simulink model "Quadcopter_Dynamics_ver2"  (R2026a)
settings: Solver=VariableStepAuto  StopTime=20.0
libraries: slpidlib x1
settings Model: Creator=aarus  LastModifiedBy=Ashwini

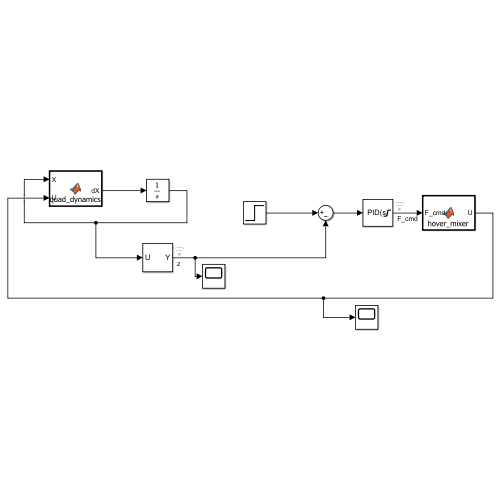
[thumbnail: Simulink's stored preview of the top-level diagram]
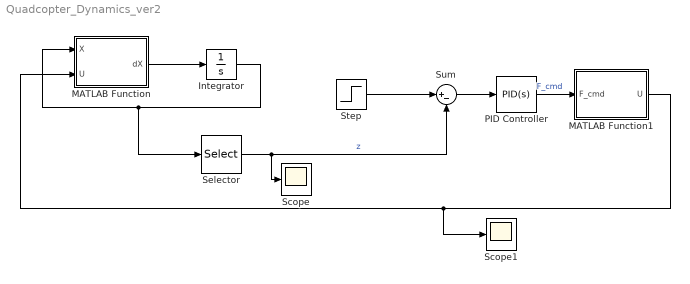
== system Quadcopter_Dynamics_ver2 ==
  Integrator : Integrator  InitialCondition=[0;0;0;0;0;0;0;0;0;0;0;0]
  MATLAB Function : MATLAB Function  TreatAsAtomicUnit=on
  MATLAB Function1 : MATLAB Function  TreatAsAtomicUnit=on
  PID Controller : slpidlib/PID Controller  Controller=PID  Form=Parallel  TimeDomain=Continuous-time  UseExternalTs=off  SampleTime=-1  IntegratorMethod=Forward Euler  FilterMethod=Forward Euler  ControllerParametersSource=internal  P=56.8136  I=7.3365  UseKiTs=off  D=31.7435  UseExternalDerivativeSource=off  N=100  UseFilter=on  TunerSelectOption=Transfer Function Based (PID Tuner App)  InitialConditionSource=internal  InitialConditionForIntegrator=0  InitialConditionForFilter=0  DifferentiatorICPrevScaledInput=0  ExternalReset=none  TrackingMode=off  Kt=1  LimitOutput=on  SatLimitsSource=internal  UpperSaturationLimit=20  LowerSaturationLimit=0  LinearizeAsGain=on  AntiWindupMode=none  Kb=1  LimitIntegrator=off  UpperIntegratorSaturationLimit=inf  LowerIntegratorSaturationLimit=-inf  POutMin=[]  POutMax=[]  IOutMin=[]  IOutMax=[]  DOutMin=[]  DOutMax=[]  NOutMin=[]  NOutMax=[]  SumOutMin=[]  SumOutMax=[]  SaturationOutMin=[]  SaturationOutMax=[]  PParamMin=[]  PParamMax=[]  IParamMin=[]  IParamMax=[]  DParamMin=[]  DParamMax=[]  NParamMin=[]  NParamMax=[]  KbParamMin=[]  KbParamMax=[]  KtParamMin=[]  KtParamMax=[]  KbOutMin=[]  KbOutMax=[]  KtOutMin=[]  KtOutMax=[]  IntegratorOutMin=[]  IntegratorOutMax=[]  FilterOutMin=[]  FilterOutMax=[]  SumI1OutMin=[]  SumI1OutMax=[]  SumI2OutMin=[]  SumI2OutMax=[]  SumI3OutMin=[]  SumI3OutMax=[]  SumI4OutMin=[]  SumI4OutMax=[]  SumDOutMin=[]  SumDOutMax=[]  DifferentiatorOutMin=[]  DifferentiatorOutMax=[]  FilterDiffOutCoefMin=[]  FilterDiffOutCoefMax=[]  ReciprocalOutMin=[]  ReciprocalOutMax=[]  SumDenOutMin=[]  SumDenOutMax=[]  SumNumOutMin=[]  SumNumOutMax=[]  DivideOutMin=[]  DivideOutMax=[]  UdiffTsProdOutMin=[]  UdiffTsProdOutMax=[]  NTsProdOutMin=[]  NTsProdOutMax=[]  UintegralTsProdOutMin=[]  UintegralTsProdOutMax=[]  UngainTsProdOutMin=[]  UngainTsProdOutMax=[]  ClampingZeroOutDataTypeStr=Inherit: Inherit via back propagation  ClampingZeroOutMin=[]  ClampingZeroOutMax=[]  FilterDenConstantOutDataTypeStr=Inherit: Inherit via back propagation  FilterDenConstantOutMin=[]  FilterDenConstantOutMax=[]  PCopyOutDataTypeStr=Inherit: Inherit via back propagation  PCopyOutMin=[]  PCopyOutMax=[]  NCopyOutDataTypeStr=Inherit: Inherit via back propagation  NCopyOutMin=[]  NCopyOutMax=[]  IntegratorContinuousStateAttributes=''  IntegratorStateMustResolveToSignalObject=off  IntegratorRTWStateStorageClass=Auto  FilterContinuousStateAttributes=''  FilterStateMustResolveToSignalObject=off  FilterRTWStateStorageClass=Auto  ParallelPVariant=InternalParameters  IdealPVariant=Disabled  IVariant=InternalParameters  DVariant=InternalParameters  IntegratorVariant=Continuous  SatVariant=Enabled  AWVariant=Passthrough  PCopyVariant=Disabled  TRVariant=Disabled  FdbkBlocksVariant=Forward  IdealPFdbkVariant=Disabled  SatFdbkVariant=Disabled  DerivativeFilterVariant=ContFilter  NVariant=InternalParameters  NCopyVariant=Disabled  FilterICVariant=InternalICsFilter  IntegratorICVariant=InternalICs  ExternalResetVariant=Disabled  TRSumVariant=Passthrough  SumFdbkVariant=Disabled  SumVariant=Sum_PID  TsampFilterVariant=InternalTs  TsampNgainVariant=Passthrough  TsampIntegralVariant=Disabled_SignalSpec  ExternalSaturationOutDataTypeStr=Inherit: Same as second input  DerivativeSourceVariant=ErrorSignal  PreIntVariant=InternalPreInt
  Scope : Scope
      settings: ActiveDisplayYMinimum=0  ActiveDisplayYMaximum=3
  Scope1 : Scope
      settings: ActiveDisplayYMinimum=-161.48199666525053  ActiveDisplayYMaximum=10000
  Selector : Selector  InputPortWidth=12  IndexOptions=Index vector (dialog)  Indices=5  OutputSizes=1
  Step : Step  Time=0  FinalValue=2  SampleTime=0
  Sum : Sum  Inputs=|+-
  wires:
  MATLAB Function/1(dX) -> Integrator/1
  Integrator/1 -> Selector/1, MATLAB Function/1(X)
  Selector/1 -> Scope/1, Sum/2  "z"
  Step/1 -> Sum/1
  Sum/1 -> PID Controller/1
  PID Controller/1 -> MATLAB Function1/1(F_cmd)  "F_cmd"
  MATLAB Function1/1(U) -> Scope1/1, MATLAB Function/2(U)

== matlab function Quadcopter_Dynamics_ver2/MATLAB Function ==
  data: X input; dX output; U input
function dX = quad_dynamics(X, U)
    % X: 12x1 state vector [x; x_dot; y; y_dot; z; z_dot; phi; phi_dot; theta; theta_dot; psi; psi_dot]
    % U: 4x1 control input vector [w1; w2; w3; w4] (rotor speeds in rad/s)
    
    % Table 1 Parameters
    m = 0.516; g = 9.81; l = 0.225; 
    Ixx = 4.984e-3; Iyy = 4.984e-3; Izz = 8.958e-3; 
    k = 2.996e-6; 
    b = 1.260e-7; 
    
    % Aerodynamic damping coefficients
    % Set to zero for ideal kinematics as numerical values are absent from Table 1
    Ax = 0; Ay = 0; Az = 0; 
    
    % Extract rotor speeds
    w1 = U(1); w2 = U(2); w3 = U(3); w4 = U(4);
    
    % Rotor-to-Force Mapping[cite: 2]
    F = k * (w1^2 + w2^2 + w3^2 + w4^2);
    tau_phi = l * k * (w4^2 - w2^2);
    tau_theta = l * k * (w3^2 - w1^2);
    tau_psi = b * (w1^2 - w2^2 + w3^2 - w4^2);
    
    tau_B = [tau_phi; tau_theta; tau_psi];

    % Extract states 
    x2 = X(2); x4 = X(4); x6 = X(6);
    phi = X(7); phi_dot = X(8); 
    theta = X(9); theta_dot = X(10); 
    psi = X(11); psi_dot = X(12);
    
    eta_dot = [phi_dot; theta_dot; psi_dot];
    
    % Trigonometric shorthands
    C_phi = cos(phi); S_phi = sin(phi);
    C_theta = cos(theta); S_theta = sin(theta);
    C_psi = cos(psi); S_psi = sin(psi);
    
    % Initialize output derivative vector
    dX = zeros(12,1);
    
    % Translational Equations
    dX(1) = x2;
    dX(2) = -(Ax/m)*x2 + (C_psi*S_theta*C_phi + S_psi*S_phi)*(F/m);
    dX(3) = x4;
    dX(4) = -(Ay/m)*x4 + (S_psi*S_theta*C_phi - C_psi*S_phi)*(F/m);
    
    % Z-axis with Ground Constraint
    z = X(5);
    z_ddot = -(Az/m)*x6 - g + (C_phi*C_theta)*(F/m);
    
    if z <= 0 && z_ddot < 0
        dX(5) = 0; % Hit the ground, velocity is 0
        dX(6) = 0; % Acceleration is 0
    else
        dX(5) = x6;
        dX(6) = z_ddot;
    end
    
    % Jacobian Matrix J(eta)[cite: 2]
    J11 = Ixx; J12 = 0; J13 = -Ixx*S_theta;
    J21 = 0; J22 = Iyy*C_phi^2 + Izz*S_phi^2; J23 = (Iyy - Izz)*C_phi*S_phi*C_theta;
    J31 = -Ixx*S_theta; J32 = (Iyy - Izz)*C_phi*S_phi*C_theta;
    J33 = Ixx*S_theta^2 + Iyy*S_phi^2*C_theta^2 + Izz*C_phi^2*C_theta^2;
    J = [J11 J12 J13; J21 J22 J23; J31 J32 J33];
    
    % Coriolis Matrix C(eta, eta_dot)
    C11 = 0;
    C12 = (Iyy - Izz)*(theta_dot*C_phi*S_phi + psi_dot*S_phi^2*C_theta) + (Izz - Iyy)*psi_dot*C_phi^2*C_theta - Ixx*psi_dot*C_theta;
    C13 = (Izz - Iyy)*psi_dot*C_phi*S_phi*C_theta^2;
    C21 = (Izz - Iyy)*(theta_dot*C_phi*S_phi + psi_dot*S_phi*C_theta) + (Iyy - Izz)*psi_dot*C_phi^2*C_theta + Ixx*psi_dot*C_theta;
    C22 = (Izz - Iyy)*phi_dot*C_phi*S_phi;
    C23 = -Ixx*psi_dot*S_theta*C_theta + Iyy*psi_dot*S_phi^2*S_theta*C_theta + Izz*psi_dot*C_phi^2*S_theta*C_theta;
    C31 = (Iyy - Izz)*psi_dot*C_theta^2*S_phi*C_phi - Ixx*theta_dot*C_theta;
    
    % Corrected C32 based on paper extraction
    C32 = (Izz - Iyy)*(theta_dot*C_phi*S_phi*S_theta + phi_dot*S_phi^2*C_theta) + (Iyy - Izz)*phi_dot*C_phi^2*C_theta + Ixx*psi_dot*S_theta*C_theta - Iyy*psi_dot*S_phi^2*S_theta*C_theta - Izz*psi_dot*C_phi^2*S_theta*C_theta;
    
    C33 = (Iyy - Izz)*phi_dot*C_phi*S_phi*C_theta^2 - Iyy*theta_dot*S_phi^2*C_theta*S_theta - Izz*theta_dot*C_phi^2*C_theta*S_theta + Ixx*theta_dot*C_theta*S_theta;
    C_mat = [C11 C12 C13; C21 C22 C23; C31 C32 C33];
    
    % Rotational Equations
    eta_ddot = J \ (tau_B - C_mat * eta_dot);
    
    dX(7) = phi_dot;
    dX(8) = eta_ddot(1);
    dX(9) = theta_dot;
    dX(10) = eta_ddot(2);
    dX(11) = psi_dot;
    dX(12) = eta_ddot(3);
end

== matlab function Quadcopter_Dynamics_ver2/MATLAB Function1 ==
  data: F_cmd input; U output
function U = hover_mixer(F_cmd)
    % Four equal rotor speeds for altitude-only control
    % U = [w1; w2; w3; w4], rad/s

    k = 2.996e-6; %[cite: 1]

    F_cmd = max(0, F_cmd);
    w_req = sqrt(F_cmd/(4*k));

    U = [w_req; w_req; w_req; w_req];
end
